simulink model "PV_MG_DroopMPPT_VPH_OneFarm_VariableDT_VariableSampling"  (R2015a)
settings: Solver=ode3  StartTime=0.0  StopTime=inf  FixedStep=DT  RelTol=1e-3
undefined symbols (not defined in the file): CT, DT
libraries: powerlib x25, simulink x6, powerlib_meascontrol x4, simulink_extras x1, re_lib x1
settings Model: PauseTimes=1.45  CovModelRefEnable=off  Creator=Nady  LastModifiedBy=ga63vey
settings DataIOCC: SaveFormat=StructureWithTime
settings HardwareCC: ProdBitPerPointer=64  ProdLargestAtomicFloat=Float  ProdIntDivRoundTo=Zero  ProdEndianess=LittleEndian  ProdHWDeviceType=Specified
settings GRTTargetCC: GeneratePreprocessorConditionals=Use local settings

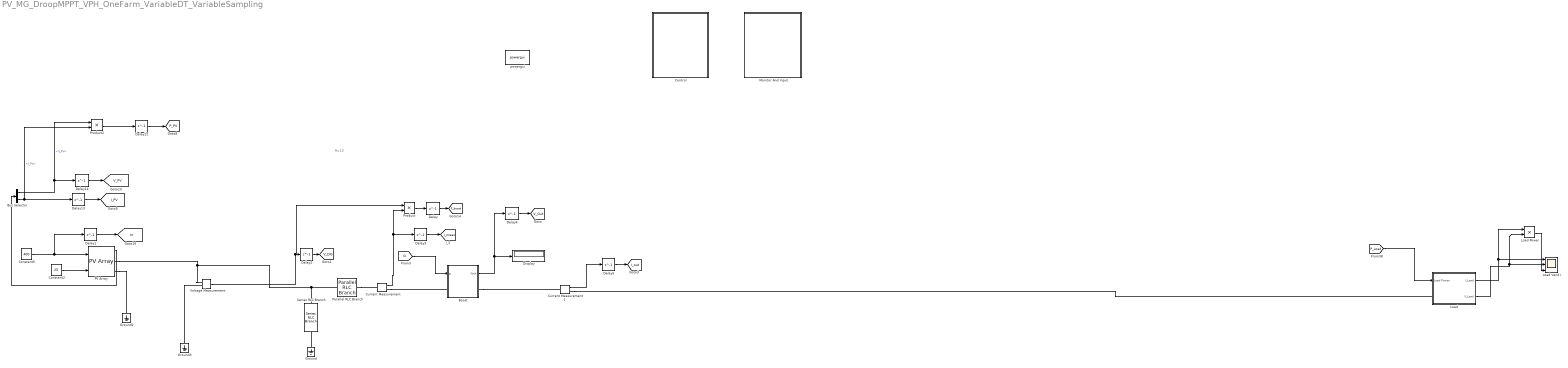
== system PV_MG_DroopMPPT_VPH_OneFarm_VariableDT_VariableSampling ==
  note: R=10
  Boost : Subsystem
  Bus Selector : BusSelector  OutputSignals=V_PV,I_PV
  Constant2 : Constant  Value=25
  Constant5 : Constant  Value=400  SampleTime=0
  "Control " : Subsystem
  Current Measurement : powerlib/Measurements/Current Measurement  PhasorSimulation=off  OutputType=Complex  PSBequivalent=0
  Current Measurement1 : powerlib/Measurements/Current Measurement  PhasorSimulation=off  OutputType=Complex  PSBequivalent=0
  Delay{,1..5,12..14} (9 alike) : Delay  DelayLength=1  InitialCondition=0
  Display : Display
  Ground : powerlib/Elements/Ground  LConnTagsString=a
  Ground2 : powerlib/Elements/Ground  LConnTagsString=a
  Ground3 : powerlib/Elements/Ground  LConnTagsString=a
  Load : Subsystem
  Load Power : Product
  Load Vand I : Scope  NumInputPorts=3
      settings: YMin=-350.25555~2.15805~-1449.82848  YMax=3150.38643~330.92882~4956.57534  SaveName=ScopeData2
  Monitor And Input : Subsystem
  PV Array : re_lib/Solar/PV Array  Npar=5  Nser=1  PlotType=one module @ 25 deg.C & specified irradiances  S_vec="[ 1000  800 ]"  Temp_C_vec=[35]  ModuleName=Sun Earth Solar Power TDB125x125-36-P 80W  PlotWhenSelected=off  Pm=80.004  Ncell=36  Voc=21.9  Isc=5  Vm=17.7  Im=4.52  beta_Voc_pc=-0.32  alpha_Isc_pc=0.04  beta_Voc=-0.07008  alpha_Isc=0.002  IL=5.0238  I0=3.6974e-11  nI=0.92596  Rsh=70.2892  Rs=0.35567  BAL=on  Tc=1e-6  Tfilter=5e-5
  Parallel RLC Branch : powerlib/Elements/Parallel RLC Branch  LConnTagsString=a  RConnTagsString=__new0  BranchType=RL  Resistance=10  Inductance=0.0164  SetiL0=off  InitialCurrent=0  Capacitance=1e-6  Setx0=off  InitialVoltage=0  Measurements=None
  Product : Product
  Product2 : Product
  Series RLC Branch : powerlib/Elements/Series RLC Branch  LConnTagsString=__new0  RConnTagsString=__new0  BranchType=C  Resistance=0.1  Inductance=1e-3  SetiL0=off  InitialCurrent=0  Capacitance=0.1  Setx0=off  InitialVoltage=0  Measurements=None
  Voltage Measurement : powerlib/Measurements/Voltage Measurement  PhasorSimulation=off  OutputType=Complex  PSBequivalent=0
  powergui : powerlib/powergui  Priority=1  SimulationMode=Discrete  SolverType=Tustin  SampleTime=DT  frequency=60  SPID=off  DisableSnubberDevices=off  DisableRonSwitches=off  DisableVfSwitches=off  SwTol=0  DisplayEquations=off  Interpol=off  methode=on  Ts=20  FunctionMessages=off  echomessages=off  HookPort=off  EnableUseOfTLC=off  x0status=blocks  frequencyindice=0  Pbase=100e6  ErrMax=1e-4  Iterations=50  UnitsV=kV  UnitsW=MW  buscounter=0  RestoreLinks=warning  ResistiveCurrentMeasurement=off  Frange=[0:2:500]  Ylog=off  Xlog=on  ShowGrid=off  save=off  variable=ZData  structure=0  ZoomFFT=off  StartTime=0.0  cycles=1  DisplayStyle=1  fundamental=60  FreqAxis=off  MaxFrequency=1000  frequencyindicesteady=1  RmsSteady=1  display=off
  tag scope: I_PV=global, I_meas=global, I_out=global, Irr=global, P_PV=global, P_boost=global, V_DG=global, V_Out=global, V_PV=global
  wires:
  Boost/1(Vout) -> Display/1, Delay4/1
  Voltage Measurement/1 -> Delay2/1, Product/1
  Current Measurement/1 -> Product/2, Delay3/1
  [P_Load] -> Load/1(Load Power)
  Load/1(I_Load) -> Load Power/1, Load Vand I/1
  Load/2(V_Load) -> Load Power/2, Load Vand I/2
  Load Power/1 -> Load Vand I/3
  Current Measurement1/1 -> Delay5/1
  Product/1 -> Delay/1
  Delay/1 -> [P_boost]
  Delay2/1 -> [V_DG]
  Delay3/1 -> [I_meas]
  Delay4/1 -> [V_Out]
  Delay5/1 -> [I_out]
  Constant2/1 -> PV Array/2
  Bus Selector/1 -> Delay14/1, Product2/1  "<V_PV>"
  Bus Selector/2 -> Delay13/1, Product2/2  "<I_PV>"
  PV Array/1 -> Bus Selector/1
  Product2/1 -> Delay12/1
  Delay12/1 -> [P_PV]
  [G] -> Boost/1(g)
  Delay13/1 -> [I_PV]
  Delay14/1 -> [V_PV]
  Constant5/1 -> Delay1/1, PV Array/1
  Delay1/1 -> [Irr]
  connections:
  Current Measurement/RConn1 -- Boost/LConn1
  Voltage Measurement/LConn1 -- PV Array/RConn1 -- Parallel RLC Branch/LConn1 -- Series RLC Branch/LConn1
  Boost/RConn1 -- Current Measurement1/LConn1
  Current Measurement1/RConn1 -- Load/LConn1
  Ground/LConn1 -- Series RLC Branch/RConn1
  PV Array/RConn2 -- Ground2/LConn1
  Voltage Measurement/LConn2 -- Ground3/LConn1
  Parallel RLC Branch/RConn1 -- Current Measurement/LConn1

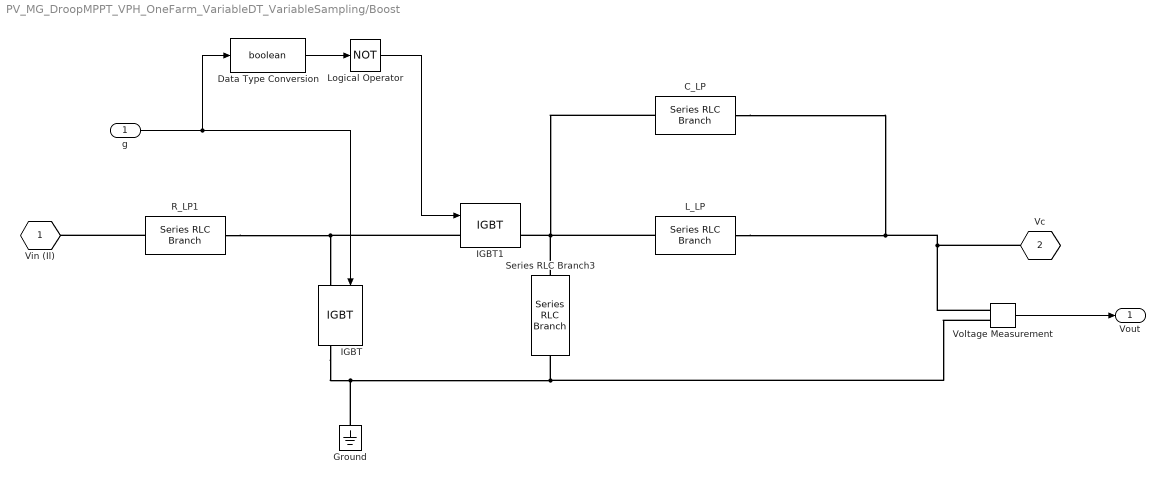
== system PV_MG_DroopMPPT_VPH_OneFarm_VariableDT_VariableSampling/Boost ==
  g : Inport
  C_LP : powerlib/Elements/Series RLC Branch  LConnTagsString=__new0  RConnTagsString=__new0  BranchType=R  Resistance=1  Inductance=1e-3  SetiL0=off  InitialCurrent=0  Capacitance=0.004  Setx0=off  InitialVoltage=0  Measurements=None
  Data Type Conversion : DataTypeConversion  OutDataTypeStr=boolean
  Ground : powerlib/Elements/Ground  LConnTagsString=a
  IGBT : powerlib/Power Electronics/IGBT  Ron=0.001  Lon=0  Vf=1  Tf=1e-6  Tt=2e-6  IC=0  Rs=1e5  Cs=inf  Measurements=on
  IGBT1 : powerlib/Power Electronics/IGBT  Ron=0.001  Lon=0  Vf=1  Tf=1e-6  Tt=2e-6  IC=0  Rs=1e5  Cs=inf  Measurements=on
  L_LP : powerlib/Elements/Series RLC Branch  LConnTagsString=__new0  RConnTagsString=__new0  BranchType=L  Resistance=0.01  Inductance=0.0164  SetiL0=off  InitialCurrent=0  Capacitance=6e-2  Setx0=off  InitialVoltage=0  Measurements=None
  Logical Operator : Logic  Operator=NOT  AllPortsSameDT=off  OutDataTypeStr=boolean
  R_LP1 : powerlib/Elements/Series RLC Branch  LConnTagsString=__new0  RConnTagsString=__new0  BranchType=L  Resistance=0.01  Inductance=7e-3  SetiL0=off  InitialCurrent=0  Capacitance=6e-2  Setx0=off  InitialVoltage=0  Measurements=None
  Series RLC Branch3 : powerlib/Elements/Series RLC Branch  LConnTagsString=__new0  RConnTagsString=__new0  BranchType=C  Resistance=0.005  Inductance=1e-3  SetiL0=off  InitialCurrent=0  Capacitance=1e-2  Setx0=off  InitialVoltage=0  Measurements=None
  Voltage Measurement : powerlib/Measurements/Voltage Measurement  PhasorSimulation=off  OutputType=Complex  PSBequivalent=0
  Vin (Il) : PMIOPort  Tag=PMCPort  Port=1  Side=Left
  Vc : PMIOPort  Tag=PMCPort  Port=2  Side=Right
  Vout : Outport
  wires:
  Voltage Measurement/1 -> Vout/1
  g/1 -> Data Type Conversion/1, IGBT/1
  Data Type Conversion/1 -> Logical Operator/1
  Logical Operator/1 -> IGBT1/1
  connections:
  IGBT/RConn1 -- Ground/LConn1 -- Voltage Measurement/LConn2 -- Series RLC Branch3/RConn1
  IGBT1/LConn1 -- R_LP1/LConn1 -- IGBT/LConn1
  R_LP1/RConn1 -- Vin (Il)/RConn1
  Vc/RConn1 -- L_LP/LConn1 -- C_LP/LConn1 -- Voltage Measurement/LConn1
  C_LP/RConn1 -- L_LP/RConn1 -- Series RLC Branch3/LConn1 -- IGBT1/RConn1

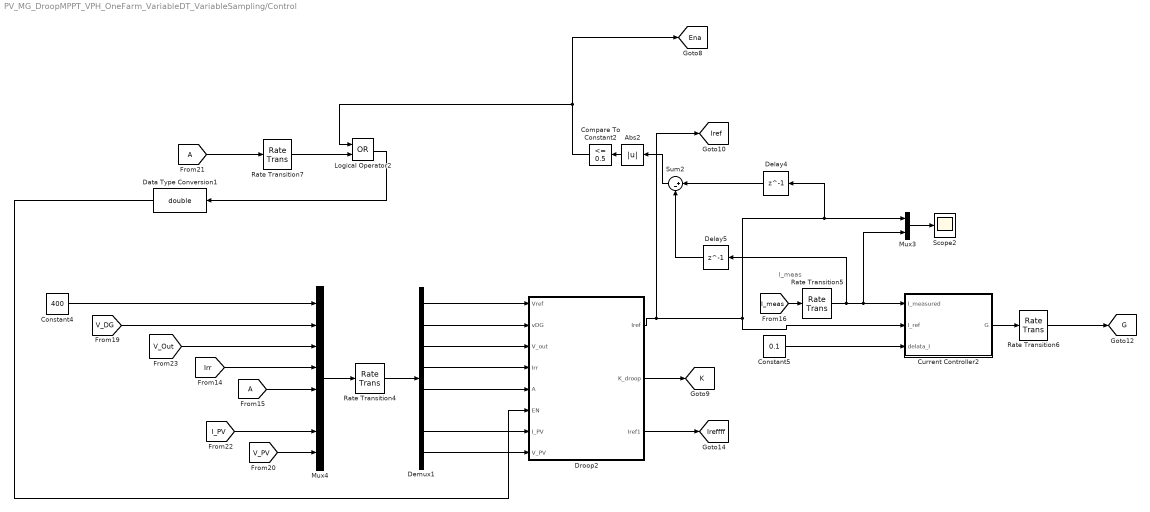
== system PV_MG_DroopMPPT_VPH_OneFarm_VariableDT_VariableSampling/Control  ==
  note: I_meas
  Abs2 : Abs
  Compare To Constant2 : simulink/Logic and Bit Operations/Compare To Constant  relop=<=  const=0.5  OutDataTypeStr=boolean
  Constant4 : Constant  Value=400  SampleTime=DT
  Constant5 : Constant  Value=0.1  SampleTime=CT
  Current Controller2 : Subsystem  TreatAsAtomicUnit=on
  Data Type Conversion1 : DataTypeConversion  OutDataTypeStr=double
  Delay4 : Delay  DelayLength=1  InitialCondition=0
  Delay5 : Delay  DelayLength=1  InitialCondition=0
  Demux1 : Demux  Outputs=8
  Droop2 : Subsystem  TreatAsAtomicUnit=on
  Logical Operator2 : Logic  Operator=OR  AllPortsSameDT=off  OutDataTypeStr=boolean
  Mux3 : Mux  Inputs=2
  Mux4 : Mux  Inputs=8
  Rate Transition4 : RateTransition  OutPortSampleTime=CT
  Rate Transition5 : RateTransition  OutPortSampleTime=CT
  Rate Transition6 : RateTransition  OutPortSampleTime=DT
  Rate Transition7 : RateTransition  OutPortSampleTime=CT
  Scope2 : Scope
      settings: YMin=-3.65633  YMax=32.86051  SaveName=ScopeData2  SampleInput=on  SampleTime=CT
  Sum2 : Sum  Inputs=|+-
  tag scope: Ena=global, G=global, Iref=global, Ireffff=global, K=global
  wires:
  Droop2/1(Iref) -> [Iref], Mux3/1, Delay4/1, Current Controller2/2(I_ref)
  [I_meas] -> Rate Transition5/1
  Constant5/1 -> Current Controller2/3(delata_I)
  Current Controller2/1(G) -> Rate Transition6/1
  Droop2/2(K_droop) -> [K]
  Mux3/1 -> Scope2/1
  Droop2/3(Iref1) -> [Ireffff]
  Sum2/1 -> Abs2/1
  Abs2/1 -> Compare To Constant2/1
  Delay4/1 -> Sum2/1
  Delay5/1 -> Sum2/2
  Constant4/1 -> Mux4/1
  [V_DG] -> Mux4/2
  [V_Out] -> Mux4/3
  [Irr] -> Mux4/4
  [A] -> Mux4/5
  [I_PV] -> Mux4/7
  [V_PV] -> Mux4/8
  Mux4/1 -> Rate Transition4/1
  Rate Transition4/1 -> Demux1/1
  Demux1/1 -> Droop2/1(Vref)
  Demux1/2 -> Droop2/2(vDG)
  Demux1/3 -> Droop2/3(V_out)
  Demux1/4 -> Droop2/4(Irr)
  Demux1/5 -> Droop2/5(A)
  Demux1/7 -> Droop2/7(I_PV)
  Demux1/8 -> Droop2/8(V_PV)
  Rate Transition5/1 -> Delay5/1, Mux3/2, Current Controller2/1(I_measured)
  Rate Transition6/1 -> [G]
  [A] -> Rate Transition7/1
  Compare To Constant2/1 -> [Ena], Logical Operator2/1
  Logical Operator2/1 -> Data Type Conversion1/1
  Data Type Conversion1/1 -> Droop2/6(EN)
  Rate Transition7/1 -> Logical Operator2/2

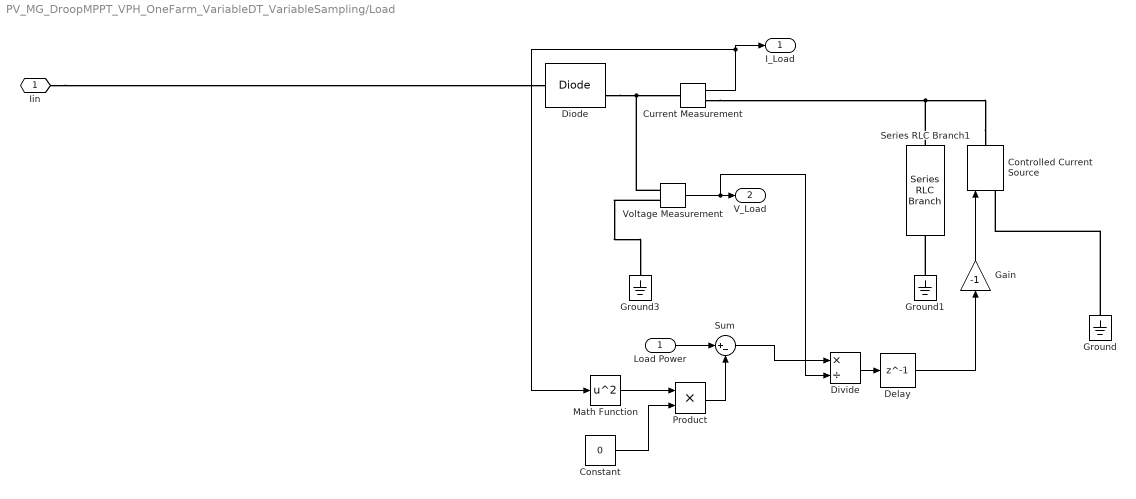
== system PV_MG_DroopMPPT_VPH_OneFarm_VariableDT_VariableSampling/Load ==
  Load Power : Inport
  Constant : Constant  Value=0
  Controlled Current Source : powerlib/Electrical Sources/Controlled Current Source  Initialize=on  Source_Type=AC  Amplitude=0  Phase=0  Frequency=0  Measurements=None
  Current Measurement : powerlib/Measurements/Current Measurement  PhasorSimulation=off  OutputType=Complex  PSBequivalent=0
  Delay : Delay  DelayLength=1  InitialCondition=0
  Diode : powerlib/Power Electronics/Diode  Ron=0.001  Lon=0  Vf=0.8  IC=0  UseSnubber=off  Rs=500  Cs=250e-9  Measurements=on
  Divide : Product  Inputs=*/
  Gain : Gain  Gain=-1
  Ground : powerlib/Elements/Ground  LConnTagsString=a
  Ground1 : powerlib/Elements/Ground  LConnTagsString=a
  Ground3 : powerlib/Elements/Ground  LConnTagsString=a
  Math Function : Math  Operator=square  SaturateOnIntegerOverflow=on
  Product : Product
  Series RLC Branch1 : powerlib/Elements/Series RLC Branch  LConnTagsString=__new0  RConnTagsString=__new0  BranchType=C  Resistance=1  Inductance=1e-3  SetiL0=off  InitialCurrent=0  Capacitance=1e-3  Setx0=off  InitialVoltage=0  Measurements=None
  Sum : Sum  Inputs=|+-
  Voltage Measurement : powerlib/Measurements/Voltage Measurement  PhasorSimulation=off  OutputType=Complex  PSBequivalent=0
  Iin : PMIOPort  Port=1  Side=Left
  I_Load : Outport
  V_Load : Outport  Port=2
  wires:
  Gain/1 -> Controlled Current Source/1
  Divide/1 -> Delay/1
  Delay/1 -> Gain/1
  Math Function/1 -> Product/1
  Constant/1 -> Product/2
  Load Power/1 -> Sum/1
  Product/1 -> Sum/2
  Sum/1 -> Divide/1
  Current Measurement/1 -> Math Function/1, I_Load/1
  Voltage Measurement/1 -> Divide/2, V_Load/1
  connections:
  Voltage Measurement/LConn1 -- Diode/RConn1 -- Current Measurement/LConn1
  Voltage Measurement/LConn2 -- Ground3/LConn1
  Ground/LConn1 -- Controlled Current Source/LConn1
  Controlled Current Source/RConn1 -- Current Measurement/RConn1 -- Series RLC Branch1/LConn1
  Ground1/LConn1 -- Series RLC Branch1/RConn1
  Iin/RConn1 -- Diode/LConn1

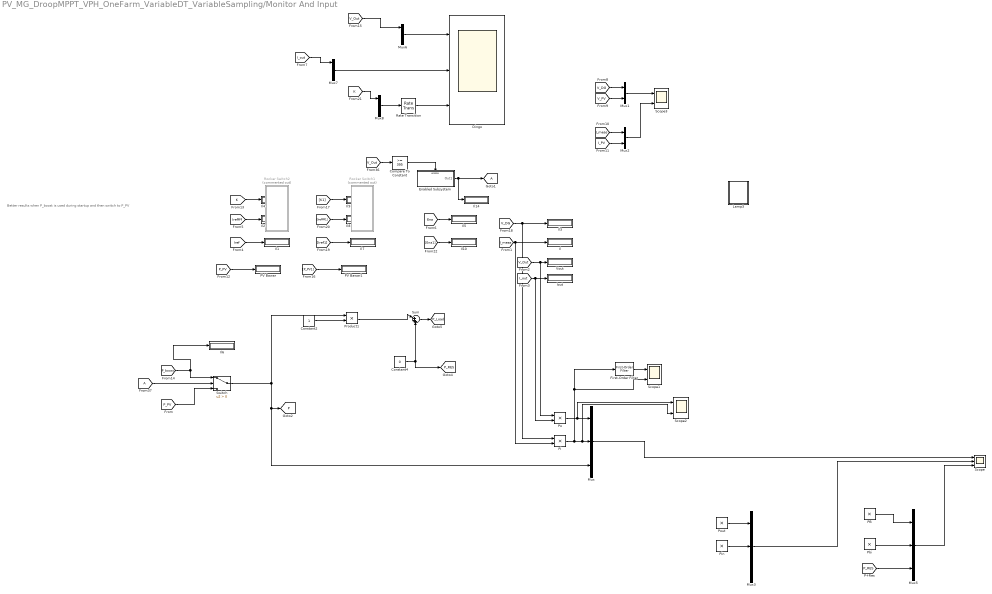
== system PV_MG_DroopMPPT_VPH_OneFarm_VariableDT_VariableSampling/Monitor And Input ==
  note: Better results when P_boost is used during startup and then switch to P_PV
  Compare To Constant : simulink/Logic and Bit Operations/Compare To Constant  relop=>=  const=395  OutDataTypeStr=boolean
  Constant2 : Constant  SampleTime=0
  Constant4 : Constant  Value=0  SampleTime=0
  Dingo : Scope  NumInputPorts=3
      settings: ShowLegends=on  TimeRange=3.8087  YMin=0~0~0  YMax=400~1.2~1.4
  Enabled Subsystem : Subsystem  TreatAsAtomicUnit=on
  First-Order Filter : powerlib_meascontrol/Filters/First-Order Filter  FilterType=Lowpass  Tc=1/400  Ts=DT  Initialize=off  Vac_Init=[0, 0, 60]  Vdc_Init=0  PlotResponse=off  FreqRange="[0,  200,  1]"
  Il{,1..10,14} (12 alike) : Display
  Iout : Display
  Lamp3 : Subsystem  DialogController=hmiCreateDDGDialog  mask(MWDashboardBlock){webBlockId=a411fb8a-8cc9-40be-9d83-47cf8fd6e8c1, webBlockType=lamp, ShowInLibBrowser=on, ShowInitialText=on, HMISrcModelName=[]}
      mask prompts: webBlockType "WebBlock Type"; HMISrcModelName "Source Model"
      mask Help: helpview([docroot '/mapfiles/simulink.map'], 'hmi_lamp')
      mask Display:
      | if strcmp(get_param(bdroot(gcb),'BlockDiagramType'), 'library')
      |     image([(matlabroot) '/toolbox/simulink/hmi/icons/Lamp.png']);
      | end
  Mux{,3,5..8} (6 alike) : Mux  Inputs=3
  Mux1 : Mux  Inputs=2
  Mux2 : Mux  Inputs=2
  PB : Product
  PV Bawar : Display
  PV Bawar1 : Display
  Pbi : Product
  Pi : Product
  Pin : Product
  Po : Product
  Pout : Product
  Product1 : Product
  Rate Transition : RateTransition  OutPortSampleTime=DT
  Rocker Switch1 : Subsystem  Commented=on  DialogController=hmiCreateDDGDialog  mask(MWDashboardBlock){webBlockId=5e99b1b3-df07-4cef-a3f6-0ddfeeb3b4e9, webBlockType=rockerswitch, ShowInLibBrowser=on, ShowInitialText=on, HMISrcModelName=[]}
      mask prompts: webBlockId "WebBlock Id"; webBlockType "WebBlock Type"; HMISrcModelName "Source Model"
      mask Help: helpview([docroot '/mapfiles/simulink.map'], 'hmi_rocker_switch')
      mask Display:
      | if strcmp(get_param(bdroot(gcb),'BlockDiagramType'), 'library')
      |     image([(matlabroot) '/toolbox/simulink/hmi/icons/RockerSwitch.png']);
      | end
  Rocker Switch2 : Subsystem  Commented=on  DialogController=hmiCreateDDGDialog  mask(MWDashboardBlock){webBlockId=5e99b1b3-df07-4cef-a3f6-0ddfeeb3b4e9, webBlockType=rockerswitch, ShowInLibBrowser=on, ShowInitialText=on, HMISrcModelName=[]}
      mask prompts: webBlockId "WebBlock Id"; webBlockType "WebBlock Type"; HMISrcModelName "Source Model"
      mask Help: helpview([docroot '/mapfiles/simulink.map'], 'hmi_rocker_switch')
      mask Display:
      | if strcmp(get_param(bdroot(gcb),'BlockDiagramType'), 'library')
      |     image([(matlabroot) '/toolbox/simulink/hmi/icons/RockerSwitch.png']);
      | end
  Scope : Scope  NumInputPorts=3
      settings: ShowLegends=on  YMin=-107.0766~-1.00000~-409.13016  YMax=623.28737~1.00000~3335.74242
  Scope1 : Scope  NumInputPorts=2
      settings: YMin=-102.309~-5  YMax=495.80827~5
  Scope2 : Scope  NumInputPorts=2
      settings: YMin=-909447.34641~-488.47375  YMax=104856.12265~844.68145  SaveName=ScopeData2
  Scope3 : Scope  NumInputPorts=2
      settings: YMin=16.5~-2  YMax=19.5~16  SaveName=ScopeData3
  Sum : Sum  Inputs=|+++
  Switch : Switch  Criteria=u2 > Threshold
  Vout : Display
  tag scope: A=global, P=global, P_Load=global, P_RES=global
  wires:
  [I_meas] -> Pi/2, Il/1
  [V_Out] -> Po/1, Vout/1
  [I_out] -> Po/2, Iout/1
  [V_DG] -> Il3/1, Pi/1
  Po/1 -> Scope2/1, Mux/1
  Pi/1 -> First-Order Filter/1, Scope1/2, Scope2/2, Mux/2
  [P_boost] -> Switch/1, Il6/1
  [P_PV] -> Switch/3
  [Iref] -> Il1/1
  [Ireffff] -> Il2/1
  Switch/1 -> [P], Mux/3, Product1/1
  Constant2/1 -> Product1/2
  [Ena] -> Il5/1
  First-Order Filter/1 -> Scope1/1
  Mux1/1 -> Scope3/1
  [V_DG] -> Mux1/1
  [V_PV] -> Mux1/2
  Mux2/1 -> Scope3/2
  [I_meas] -> Mux2/1
  [I_PV] -> Mux2/2
  [P_PV] -> PV Bawar/1
  [K] -> Il4/1
  [Iref1] -> Il7/1
  [Ireffff1] -> Il8/1
  [P_PV1] -> PV Bawar1/1
  [K1] -> Il9/1
  [Ena1] -> Il10/1
  Pout/1 -> Mux3/1
  Pin/1 -> Mux3/2
  Product1/1 -> Sum/1
  Sum/1 -> [P_Load]
  Constant4/1 -> Sum/3, [P_RES]
  Mux/1 -> Scope/1
  Mux3/1 -> Scope/2
  PB/1 -> Mux5/1
  Pbi/1 -> Mux5/2
  [P_RES] -> Mux5/3
  Mux5/1 -> Scope/3
  Rate Transition/1 -> Dingo/3
  [V_Out] -> Mux6/1
  Mux6/1 -> Dingo/1
  [I_out] -> Mux7/1
  Mux7/1 -> Dingo/2
  [K] -> Mux8/1
  Mux8/1 -> Rate Transition/1
  Enabled Subsystem/1(Out1) -> Il14/1, [A]
  [V_Out] -> Compare To Constant/1
  Compare To Constant/1 -> Enabled Subsystem/Enable
  [A] -> Switch/2

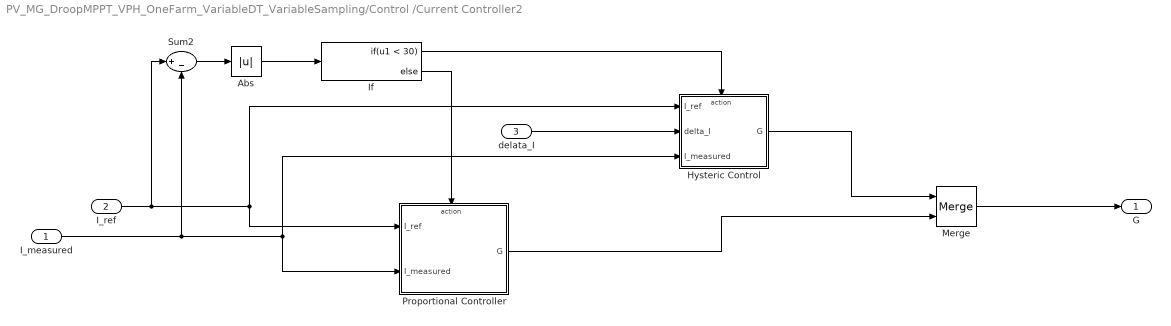
== system PV_MG_DroopMPPT_VPH_OneFarm_VariableDT_VariableSampling/Control /Current Controller2 ==
  I_measured : Inport  SampleTime=CT
  I_ref : Inport  Port=2  SampleTime=CT
  delata_I : Inport  Port=3
  Abs : Abs
  Hysteric Control : Subsystem  TreatAsAtomicUnit=on
  If : If  IfExpression=u1 < 30
  Merge : Merge
  Proportional Controller : Subsystem  TreatAsAtomicUnit=on
  Sum2 : Sum  Inputs=|+-
  G : Outport
  wires:
  Merge/1 -> G/1
  Abs/1 -> If/1
  Sum2/1 -> Abs/1
  Hysteric Control/1(G) -> Merge/1
  delata_I/1 -> Hysteric Control/2(delta_I)
  Proportional Controller/1(G) -> Merge/2
  I_measured/1 -> Sum2/2, Proportional Controller/2(I_measured), Hysteric Control/3(I_measured)
  I_ref/1 -> Proportional Controller/1(I_ref), Hysteric Control/1(I_ref), Sum2/1
  If/2 -> Proportional Controller/Action
  If/1 -> Hysteric Control/Action

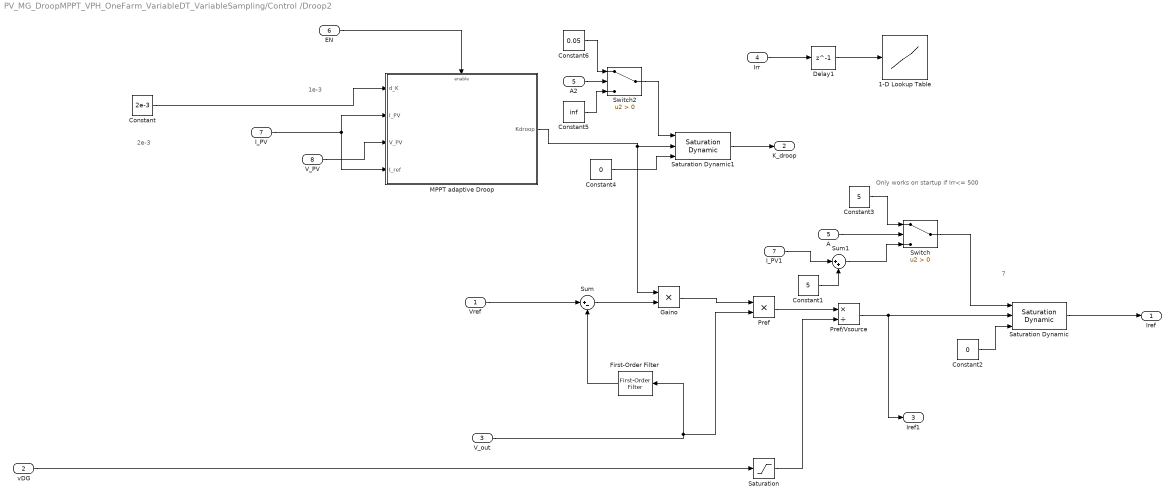
== system PV_MG_DroopMPPT_VPH_OneFarm_VariableDT_VariableSampling/Control /Droop2 ==
  note: Only works on startup if Irr<= 500
  note: 2e-3
  note: 7
  note: 1e-3
  Vref : Inport  SampleTime=CT
  vDG : Inport  Port=2  SampleTime=CT
  V_out : Inport  Port=3  SampleTime=CT
  Irr : Inport  Port=4
  A : Inport  Port=5  SampleTime=CT
  EN : Inport  Port=6
  I_PV : Inport  Port=7  SampleTime=CT
  V_PV : Inport  Port=8
  1-D Lookup Table : Lookup_n-D  NumberOfTableDimensions=1  BreakpointsForDimension1=fliplr([1000 900 800 600 500 400 300 200 100 0])  Table=fliplr([17 16.5 15 14.5 11 8 2.5 2 1.5 0])  InternalRulePriority=Speed  RndMeth=Simplest  InputSameDT=on
  A2 : InportShadow  Port=5  SampleTime=CT
  Constant : Constant  Value=2e-3  SampleTime=CT
  Constant1 : Constant  Value=5  SampleTime=CT
  Constant2 : Constant  Value=0  SampleTime=CT
  Constant3 : Constant  Value=5  SampleTime=CT
  Constant4 : Constant  Value=0  SampleTime=CT
  Constant5 : Constant  Value=inf  SampleTime=CT
  Constant6 : Constant  Value=0.05  SampleTime=CT
  Delay1 : Delay  DelayLength=1  InitialCondition=0
  First-Order Filter : powerlib_meascontrol/Filters/First-Order Filter  FilterType=Lowpass  Tc=1/8000  Ts=CT  Initialize=off  Vac_Init=[0, 0, 60]  Vdc_Init=0  PlotResponse=off  FreqRange="[0,  5000,  1]"
  Gaino : Product
  I_PV1 : InportShadow  Port=7  SampleTime=CT
  MPPT adaptive Droop : Subsystem  TreatAsAtomicUnit=on
  Pref : Product
  Pref/Vsource : Product  Inputs=*/
  Saturation : Saturate  UpperLimit=inf  LowerLimit=1
  Saturation Dynamic : simulink/Discontinuities/Saturation Dynamic  OutMin=[]  OutMax=[]  OutDataTypeStr=Inherit: Same as second input  OutDataType=fixdt(1, 16)  OutScaling=2^-10  DoSatur=off
  Saturation Dynamic1 : simulink/Discontinuities/Saturation Dynamic  OutMin=[]  OutMax=[]  OutDataTypeStr=Inherit: Same as second input  OutDataType=fixdt(1, 16)  OutScaling=2^-10  DoSatur=off
  Sum : Sum  Inputs=|+-
  Sum1 : Sum  Inputs=|++
  Switch : Switch  Criteria=u2 > Threshold
  Switch2 : Switch  Criteria=u2 > Threshold
  Iref : Outport  SampleTime=CT
  K_droop : Outport  Port=2
  Iref1 : Outport  Port=3
  wires:
  MPPT adaptive Droop/1(Kdroop) -> Saturation Dynamic1/2, Gaino/1
  I_PV/1 -> MPPT adaptive Droop/2(I_PV), MPPT adaptive Droop/4(I_ref)
  V_PV/1 -> MPPT adaptive Droop/3(V_PV)
  EN/1 -> MPPT adaptive Droop/Enable
  vDG/1 -> Saturation/1
  Constant/1 -> MPPT adaptive Droop/1(d_K)
  A/1 -> Switch/2
  Sum1/1 -> Switch/3
  Switch/1 -> Saturation Dynamic/1
  Irr/1 -> Delay1/1
  Delay1/1 -> 1-D Lookup Table/1
  Constant2/1 -> Saturation Dynamic/3
  Vref/1 -> Sum/1
  V_out/1 -> First-Order Filter/1, Pref/2
  Pref/Vsource/1 -> Iref1/1, Saturation Dynamic/2
  Gaino/1 -> Pref/1
  Saturation/1 -> Pref/Vsource/2
  Pref/1 -> Pref/Vsource/1
  First-Order Filter/1 -> Sum/2
  Sum/1 -> Gaino/2
  Saturation Dynamic1/1 -> K_droop/1
  Switch2/1 -> Saturation Dynamic1/1
  A2/1 -> Switch2/2
  Constant4/1 -> Saturation Dynamic1/3
  Constant5/1 -> Switch2/3
  Constant6/1 -> Switch2/1
  I_PV1/1 -> Sum1/1
  Constant1/1 -> Sum1/2
  Saturation Dynamic/1 -> Iref/1
  Constant3/1 -> Switch/1

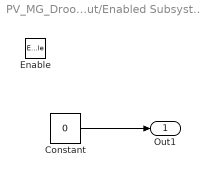
== system PV_MG_DroopMPPT_VPH_OneFarm_VariableDT_VariableSampling/Monitor And Input/Enabled Subsystem ==
  Enable : EnablePort
  Constant : Constant  Value=0
  Out1 : Outport  InitialOutput=1
  wires:
  Constant/1 -> Out1/1

== system PV_MG_DroopMPPT_VPH_OneFarm_VariableDT_VariableSampling/Monitor And Input/Lamp3 ==

== system PV_MG_DroopMPPT_VPH_OneFarm_VariableDT_VariableSampling/Monitor And Input/Rocker Switch1 ==

== system PV_MG_DroopMPPT_VPH_OneFarm_VariableDT_VariableSampling/Monitor And Input/Rocker Switch2 ==

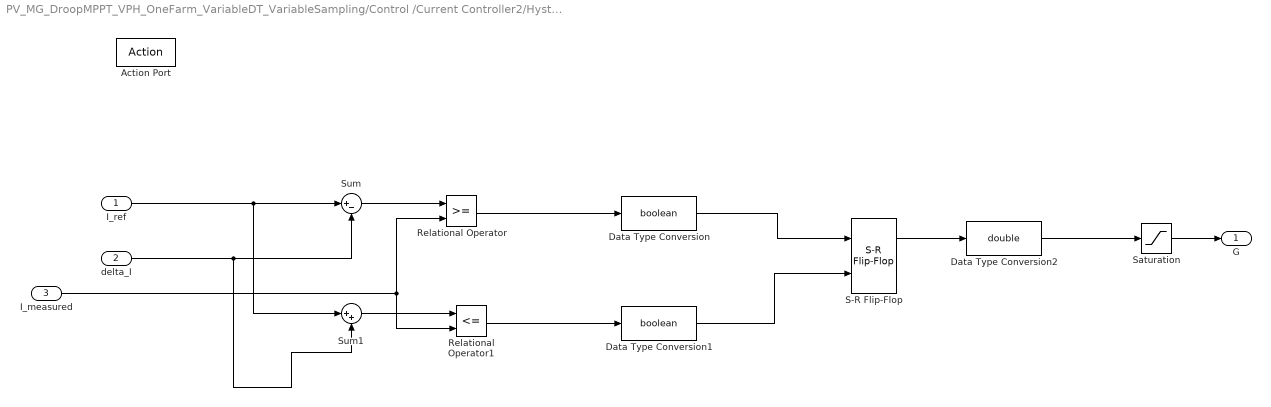
== system PV_MG_DroopMPPT_VPH_OneFarm_VariableDT_VariableSampling/Control /Current Controller2/Hysteric Control ==
  I_ref : Inport
  delta_I : Inport  Port=2
  I_measured : Inport  Port=3
  Action Port : ActionPort  ActionType=then
  Data Type Conversion : DataTypeConversion  OutDataTypeStr=boolean
  Data Type Conversion1 : DataTypeConversion  OutDataTypeStr=boolean
  Data Type Conversion2 : DataTypeConversion  OutDataTypeStr=double
  Relational Operator : RelationalOperator  OutDataTypeStr=boolean  ZeroCross=off
  Relational Operator1 : RelationalOperator  Operator=<=  OutDataTypeStr=boolean  ZeroCross=off
  S-R Flip-Flop : simulink_extras/Flip Flops/S-R Flip-Flop  initial_condition=0
  Saturation : Saturate  UpperLimit=1  LowerLimit=0
  Sum : Sum  Inputs=|+-
  Sum1 : Sum  Inputs=|++
  G : Outport
  wires:
  S-R Flip-Flop/1 -> Data Type Conversion2/1
  Saturation/1 -> G/1
  Data Type Conversion2/1 -> Saturation/1
  I_measured/1 -> Relational Operator1/2, Relational Operator/2
  Sum1/1 -> Relational Operator1/1
  Relational Operator1/1 -> Data Type Conversion1/1
  Relational Operator/1 -> Data Type Conversion/1
  Sum/1 -> Relational Operator/1
  Data Type Conversion1/1 -> S-R Flip-Flop/2
  Data Type Conversion/1 -> S-R Flip-Flop/1
  delta_I/1 -> Sum1/2, Sum/2
  I_ref/1 -> Sum/1, Sum1/1

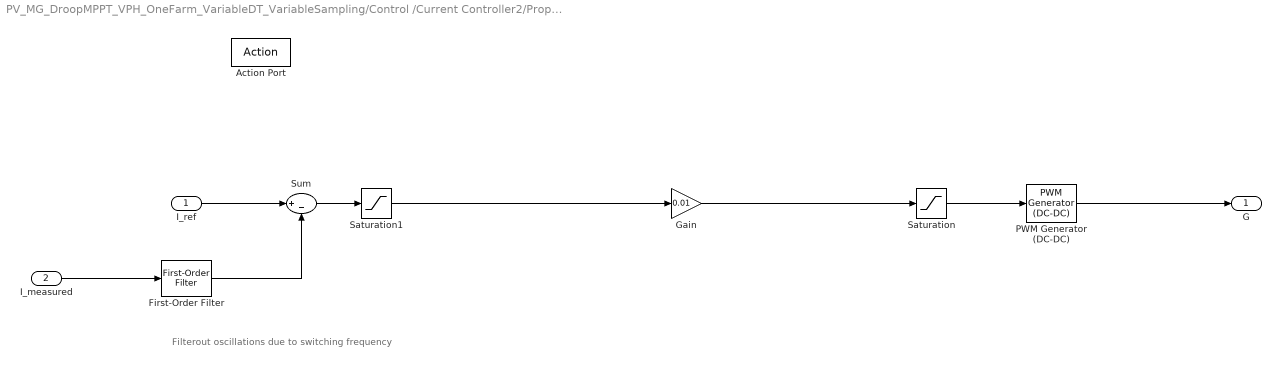
== system PV_MG_DroopMPPT_VPH_OneFarm_VariableDT_VariableSampling/Control /Current Controller2/Proportional Controller ==
  note: Filterout oscillations due to switching frequency
  I_ref : Inport
  I_measured : Inport  Port=2
  Action Port : ActionPort  ActionType=else
  First-Order Filter : powerlib_meascontrol/Filters/First-Order Filter  FilterType=Lowpass  Tc=1/8000  Ts=CT  Initialize=off  Vac_Init=[0, 0, 60]  Vdc_Init=0  PlotResponse=off  FreqRange="[0,  5000,  1]"
  Gain : Gain  Gain=0.01
  PWM Generator (DC-DC) : powerlib_meascontrol/Pulse & Signal Generators/PWM Generator (DC-DC)  Fsw=10000  Ts=CT
  Saturation : Saturate  UpperLimit=0.8  LowerLimit=0
  Saturation1 : Saturate  UpperLimit=100  LowerLimit=-100
  Sum : Sum  Inputs=|+-
  G : Outport
  wires:
  Gain/1 -> Saturation/1
  First-Order Filter/1 -> Sum/2
  I_measured/1 -> First-Order Filter/1
  Saturation1/1 -> Gain/1
  Sum/1 -> Saturation1/1
  PWM Generator (DC-DC)/1 -> G/1
  Saturation/1 -> PWM Generator (DC-DC)/1
  I_ref/1 -> Sum/1

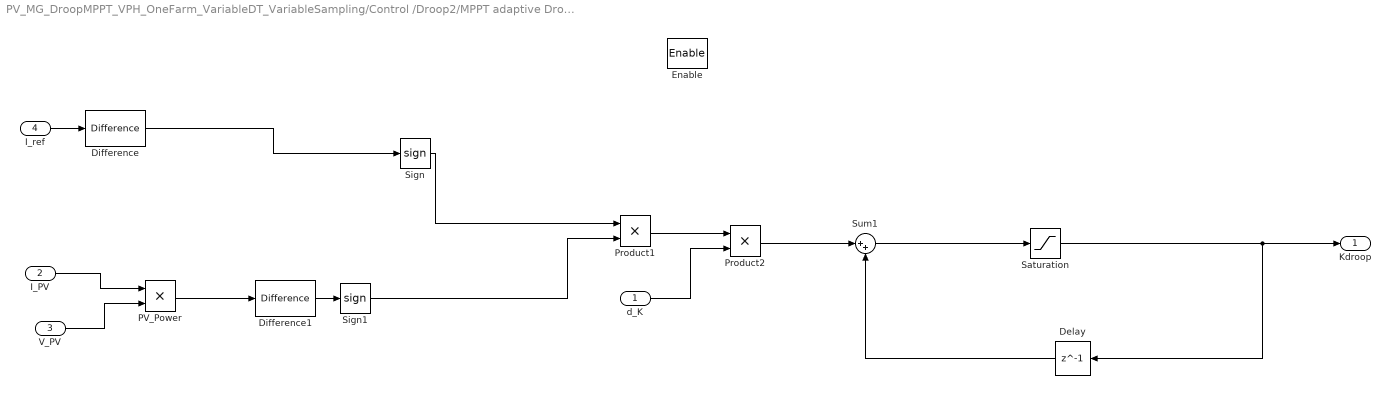
== system PV_MG_DroopMPPT_VPH_OneFarm_VariableDT_VariableSampling/Control /Droop2/MPPT adaptive Droop ==
  d_K : Inport  SampleTime=CT
  I_PV : Inport  Port=2  SampleTime=CT
  V_PV : Inport  Port=3  SampleTime=CT
  I_ref : Inport  Port=4  SampleTime=CT
  Enable : EnablePort
  Delay : Delay  DelayLength=1  InitialCondition=0  SampleTime=CT
  Difference : simulink/Discrete/Difference  ICPrevInput=0.0  InputProcessing=Inherited  OutMin=[]  OutMax=[]  OutDataType=fixdt(1, 16)  OutScaling=2^-10  DoSatur=off
  Difference1 : simulink/Discrete/Difference  ICPrevInput=0.0  InputProcessing=Inherited  OutMin=[]  OutMax=[]  OutDataType=fixdt(1, 16)  OutScaling=2^-10  DoSatur=off
  PV_Power : Product
  Product1 : Product
  Product2 : Product
  Saturation : Saturate  UpperLimit=4  LowerLimit=0
  Sign : Signum
  Sign1 : Signum
  Sum1 : Sum  Inputs=|++
  Kdroop : Outport  SampleTime=CT  InitialOutput=0.01
  wires:
  I_ref/1 -> Difference/1
  V_PV/1 -> PV_Power/2
  I_PV/1 -> PV_Power/1
  Difference/1 -> Sign/1
  Sum1/1 -> Saturation/1
  Delay/1 -> Sum1/2
  Product2/1 -> Sum1/1
  d_K/1 -> Product2/2
  Product1/1 -> Product2/1
  Sign1/1 -> Product1/2
  Difference1/1 -> Sign1/1
  PV_Power/1 -> Difference1/1
  Saturation/1 -> Delay/1, Kdroop/1
  Sign/1 -> Product1/1
